simulink model "lab3_z"  (R2013b)
settings: Solver=ode45  SolverMode=SingleTasking  StartTime=0.0  StopTime=t_max  MaxStep=0.1  RelTol=1e-3
undefined symbols (not defined in the file): d, Lo, Lrz, Mo, Mrz, t0, y0
settings Model: CovMetricSettings=dwe  CovHtmlReporting=off  covSaveCumulativeToWorkspaceVar=off  CovSaveSingleToWorkspaceVar=off  CovExternalEMLEnable=on  Creator=lev  LastModifiedBy=lev
settings DataIOCC: LimitDataPoints=off  SaveFormat=StructureWithTime
settings DebuggingCC: UnderspecifiedInitializationDetection=Simplified  MergeDetectMultiDrivingBlocksExec=error  SolverPrmCheckMsg=none  FrameProcessingCompatibilityMsg=error  SFUnexpectedBacktrackingDiag=error  SFNoUnconditionalDefaultTransitionDiag=error
settings HardwareCC: ProdBitPerPointer=64  ProdLargestAtomicFloat=Float  ProdIntDivRoundTo=Zero  ProdEndianess=LittleEndian  ProdHWDeviceType=Specified
settings ModelReferenceCC: PropagateSignalLabelsOutOfModel=on
settings SFSimCC: SimUseLocalCustomCode=on
settings RTWCC: RTWUseLocalCustomCode=on
settings GRTTargetCC: CodeReplacementLibrary=C99 (ISO)  GeneratePreprocessorConditionals=Use local settings

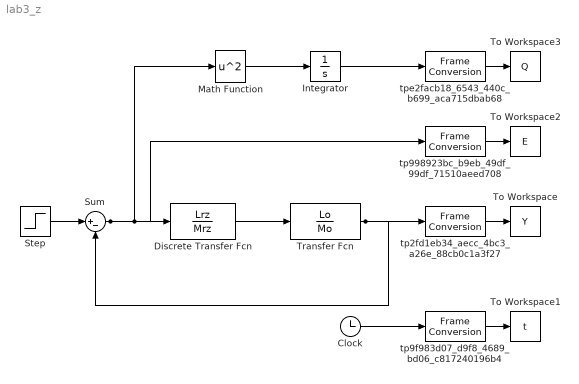
== system lab3_z ==
  Clock : Clock
  Discrete Transfer Fcn : DiscreteTransferFcn  Numerator=Lrz  Denominator=Mrz  SampleTime=d
  Integrator : Integrator
  Math Function : Math  Operator=square  SaturateOnIntegerOverflow=on
  Step : Step  Time=t0  After=y0  SampleTime=0
  Sum : Sum  Inputs=|+-
  To Workspace : ToWorkspace  VariableName=Y  SampleTime=-1
  To Workspace1 : ToWorkspace  VariableName=t  SampleTime=-1
  To Workspace2 : ToWorkspace  VariableName=E  SampleTime=-1
  To Workspace3 : ToWorkspace  VariableName=Q  SampleTime=-1
  Transfer Fcn : TransferFcn  Numerator=Lo  Denominator=Mo
  tp2fd1eb34_aecc_4bc3_a26e_88cb0c1a3f27 : FrameConversion  OutFrame=Sample-based
  tp998923bc_b9eb_49df_99df_71510aeed708 : FrameConversion  OutFrame=Sample-based
  tp9f983d07_d9f8_4689_bd06_c817240196b4 : FrameConversion  OutFrame=Sample-based
  tpe2facb18_6543_440c_b699_aca715dbab68 : FrameConversion  OutFrame=Sample-based
  wires:
  Transfer Fcn/1 -> Sum/2, tp2fd1eb34_aecc_4bc3_a26e_88cb0c1a3f27/1
  Sum/1 -> Discrete Transfer Fcn/1, Math Function/1, tp998923bc_b9eb_49df_99df_71510aeed708/1
  Step/1 -> Sum/1
  Math Function/1 -> Integrator/1
  Discrete Transfer Fcn/1 -> Transfer Fcn/1
  tp2fd1eb34_aecc_4bc3_a26e_88cb0c1a3f27/1 -> To Workspace/1
  Clock/1 -> tp9f983d07_d9f8_4689_bd06_c817240196b4/1
  tp9f983d07_d9f8_4689_bd06_c817240196b4/1 -> To Workspace1/1
  tp998923bc_b9eb_49df_99df_71510aeed708/1 -> To Workspace2/1
  Integrator/1 -> tpe2facb18_6543_440c_b699_aca715dbab68/1
  tpe2facb18_6543_440c_b699_aca715dbab68/1 -> To Workspace3/1
